simulink model "testFVOPID"  (R2020a)
settings: Solver=VariableStepAuto  StartTime=0.0  StopTime=50  RelTol=1e-3
settings Model: Creator=dell-wi  LastModifiedBy=Pio
settings DataIOCC: ReturnWorkspaceOutputs=off
settings DebuggingCC: ArithmeticOperatorsInVariantConditions=warning
settings SFSimCC: SimUseLocalCustomCode=off  CustomCodeUndefinedFunction=UseInterfaceOnly
settings RTWCC: RTWUseLocalCustomCode=off

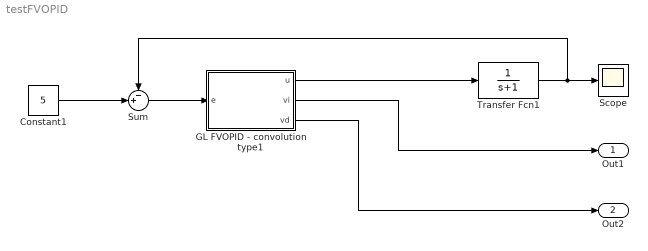
== system testFVOPID ==
  Constant1 : Constant  Value=5
  GL FVOPID - convolution type1 : Subsystem  mask{kp=1, ki=1, kd=1, sampleTime=0.01, inputBufferSize=-1, satEnab=off, satHigh=inf, satLow=-inf, integralOrderTypePopup=User defined expression, constantIntegralOrder=1, integralErrorToSetpointRatio=off, integralErrorValuesVector=[0.8, 0.6, 0.4, 0.2], integralOrderValuesVector=[1, 2, 3, 4, 5], timeDependentIntegralOrderExpression=0.1*t, derivativeOrderTypePopup=User defined expression, constantDerivativeOrder=1, derivativeErrorToSetpointRatio=off, derivativeErrorValuesVector=[0], derivativeOrderValuesVector=[1, 1], timeDependentDerivativeOrderExpression=0.1*t}
      mask prompts: kp "Proportional (P)"; ki "Integral (I)"; kd "Derivative (D)"; sampleTime "Sample time"; inputBufferSize "Input buffer size (-1 for automatically calculated)"; satEnab "Limit output"; satHigh "Upper limit"; satLow "Lower limit"; integralOrderTypePopup "Integral order type"; constantIntegralOrder "Integral order"; integralErrorToSetpointRatio "Use error/setpoint ratio"; integralErrorValuesVector "Vector of control error values"; integralOrderValuesVector "Vector of order values"; derivativeOrderTypePopup "Derivative order type"; constantDerivativeOrder "Derivative order"; derivativeErrorToSetpointRatio "Use error/setpoint ratio"; derivativeErrorValuesVector "Vector of control error values"; derivativeOrderValuesVector "Vector of order values"
      mask init:
      | % Initialize block parameters
      | fvopidToolbox.library.utils.initializeBasicModelParameters(sampleTime, inputBufferSize,'fvopidConv');
      | integralOrderTypeComboBoxValue = get_param(gcb,'integralOrderTypePopup');
      | derivativeOrderTypeComboBoxValue = get_param(gcb,'derivativeOrderTypePopup');
      | 
      | % Set order function type
      | switch integralOrderTypeComboBoxValue
      |     case 'Constant order'
      |         integralOrderType = 1;
      |     case 'Control error function'
      |         integralErrorToSetpointRatioValue = get_param(gcb,'integralErrorToSetpointRatio');
      |         if strcmp(integralErrorToSetpointRatioValue, 'on')
      |             integralOrderType = 3;
      |         else
      |             integralOrderType = 2;
      |         end
      |     otherwise
      |         integralOrderExpressionCode = get_param(gcb,'timeDependentIntegralOrderExpression');
      |         newScript = sprintf(['function y = integralTimeDependentMatlabFunction(t, e)\n'...
      |             'y = '  integralOrderExpressionCode ';\nend']);
      |         fvopidToolbox.utils.updateMatlabFunctionBlockScript('integralTimeDependentBlock', newScript,...
      |             [gcb '/integralTimeDependentSubsystem/integralTimeDependentBlock']);
      |         integralOrderType = 4;
      | end
      | 
      | switch derivativeOrderTypeComboBoxValue
      |     case 'Constant order'
      |         derivativeOrderType = 1;
      |     case 'Control error function'
      |         derivatieErrorToSetpointRatioValue = get_param(gcb,'derivativeErrorToSetpointRatio');
      |         if strcmp(derivatieErrorToSetpointRatioValue, 'on')
      |             derivativeOrderType = 3;
      |         else
      |             derivativeOrderType = 2;
      |         end
      |     otherwise
      |         derivativeOrderExpressionCode = get_param(gcb,'timeDependentDerivativeOrderExpression');
      |         newScript = sprintf(['function y = derivativeTimeDependentMatlabFunction(t, e)\n'...
      |             'y = ' derivativeOrderExpressionCode ';\nend']);
      |         fvopidToolbox.utils.updateMatlabFunctionBlockScript('derivativeTimeDependentBlock', newScript,...
      |             [gcb '/derivativeTimeDependentSubsystem/derivativeTimeDependentBlock']);
      |         derivativeOrderType = 4;
      | end
      | 
      | % Update the input ports
      | setpointInputBlock = find_system(gcb,...
      |     'LookUnderMasks','on',...
      |     'FollowLinks','on','Name','setpointInput');
      | if integralOrderType == 3 || derivativeOrderType == 3
      |     if isempty(setpointInputBlock)
      |         add_block('built-in/Inport',[gcb,'/setpointInput']);  
      |     else
      |         h = get_param([gcb '/setpointInput'], 'LineHandles'); 
      |         delete_line(h.Outport(1));
      |     end
      | 
      |     if integralOrderType == 3
      |         add_line(gcb,'setpointInput/1','integralRatioDependentSubsystem/2');
      |     end
      | 
      |     if derivativeOrderType == 3
      |         add_line(gcb,'setpointInput/1','derivativeRatioDependentSubsystem/2');
      |     end
      | else
      |     if ~isempty(setpointInputBlock)
      |         h = get_param([gcb '/setpointInput'], 'LineHandles'); 
      |         delete_line(h.Outport(1));
      |         delete_block(setpointInputBlock);
      |     end
      | end
      settings: CopyFcn=set_param(gcbh, 'LinkStatus', 'none');
      mask Callback satEnab:
      | limitOutputCheckBoxValue = get_param(gcb,'satEnab');
      | if strcmp(limitOutputCheckBoxValue, 'on')
      |    fvopidToolbox.library.utils.setMaskParameterPropertyValue('satHigh', 'MaskEnables', 'on');
      |    fvopidToolbox.library.utils.setMaskParameterPropertyValue('satLow', 'MaskEnables', 'on');
      | else
      |    fvopidToolbox.library.utils.setMaskParameterPropertyValue('satHigh', 'MaskEnables', 'off');
      |    fvopidToolbox.library.utils.setMaskParameterPropertyValue('satLow', 'MaskEnables', 'off');
      | end
      mask TypeOptions integralOrderTypePopup: Constant order | Function of control error | User defined expression
      mask Callback integralOrderTypePopup:
      | selectedComboBoxValue = get_param(gcb,'integralOrderTypePopup');
      | 
      | switch selectedComboBoxValue
      |     case 'Constant order'
      |         fvopidToolbox.library.utils.setMaskElementVisiblePropertyValue('constantIntegralOrderPanel', 'on');
      |         fvopidToolbox.library.utils.setMaskElementVisiblePropertyValue('controlErrorDependentIntegralOrderPanel', 'off');
      |         fvopidToolbox.library.utils.setMaskElementVisiblePropertyValue('timeDependentIntegralOrderPanel', 'off');
      |     case 'Control error function'
      |         fvopidToolbox.library.utils.setMaskElementVisiblePropertyValue('constantIntegralOrderPanel', 'off');
      |         fvopidToolbox.library.utils.setMaskElementVisiblePropertyValue('controlErrorDependentIntegralOrderPanel', 'on');
      |         fvopidToolbox.library.utils.setMaskElementVisiblePropertyValue('timeDependentIntegralOrderPanel', 'off');
      |     otherwise
      |         fvopidToolbox.library.utils.setMaskElementVisiblePropertyValue('constantIntegralOrderPanel', 'off');
      |         fvopidToolbox.library.utils.setMaskElementVisiblePropertyValue('controlErrorDependentIntegralOrderPanel', 'off');
      |         fvopidToolbox.library.utils.setMaskElementVisiblePropertyValue('timeDependentIntegralOrderPanel', 'on');
      | end
      mask TypeOptions derivativeOrderTypePopup: Constant order | Function of control error | User defined expression
      mask Callback derivativeOrderTypePopup:
      | selectedComboBoxValue = get_param(gcb,'derivativeOrderTypePopup');
      | 
      | switch selectedComboBoxValue
      |     case 'Constant order'
      |         fvopidToolbox.library.utils.setMaskElementVisiblePropertyValue('constantDerivativeOrderPanel', 'on');
      |         fvopidToolbox.library.utils.setMaskElementVisiblePropertyValue('controlErrorDependentDerivativeOrderPanel', 'off');
      |         fvopidToolbox.library.utils.setMaskElementVisiblePropertyValue('timeDependentDerivativeOrderPanel', 'off');
      |     case 'Control error function'
      |         fvopidToolbox.library.utils.setMaskElementVisiblePropertyValue('constantDerivativeOrderPanel', 'off');
      |         fvopidToolbox.library.utils.setMaskElementVisiblePropertyValue('controlErrorDependentDerivativeOrderPanel', 'on');
      |         fvopidToolbox.library.utils.setMaskElementVisiblePropertyValue('timeDependentDerivativeOrderPanel', 'off');
      |     otherwise
      |         fvopidToolbox.library.utils.setMaskElementVisiblePropertyValue('constantDerivativeOrderPanel', 'off');
      |         fvopidToolbox.library.utils.setMaskElementVisiblePropertyValue('controlErrorDependentDerivativeOrderPanel', 'off');
      |         fvopidToolbox.library.utils.setMaskElementVisiblePropertyValue('timeDependentDerivativeOrderPanel', 'on');
      | end
      mask DialogControl mainTab Prompt: Main
      mask DialogControl controllerParametersGroupBox Prompt: Controller parameters
      mask DialogControl outputSaturationTab Prompt: Output saturation
      mask DialogControl outputSaturationGroupBox Prompt: Output saturation
      mask DialogControl integralOrderTab Prompt: Integral order
      mask DialogControl errorDependentIntegralOrderDescription1 Prompt: Provide a vector of control error values and a vector of order vales. Vector of order values should have one element more than the vector of error. E.g. for if the vector of order values is: [e1, e2, e3] and the vector of orders is [o1, o2, o3, o4], then the orders are generated according to the following rule:
      mask DialogControl errorDependentIntegralOrderDescription2 Prompt: - order = o1 for errors > e1,
      mask DialogControl errorDependentIntegralOrderDescription3 Prompt: - order = o2 for e2 < error <= e1,
      mask DialogControl errorDependentIntegralOrderDescription4 Prompt: - order = o3 for e3 < error <= e2,
      mask DialogControl errorDependentIntegralOrderDescription5 Prompt: - order = o4 for error < e3.
      mask DialogControl timeDependentIntegralOrderDescription1 Prompt: Insert short expression which returns value of order as a function of time (t) and/or control error (e), e.g.: '2*t + e' (where 't' is current simulation time and 'e' is current value of the control error).
      mask DialogControl derivativeOrderTab Prompt: Derivative order
      mask DialogControl errorDependentDerivativeOrderDescription1 Prompt: Provide a vector of control error values and a vector of order vales. Vector of order values should have one element more than the vector of error. E.g. for if the vector of order values is: [e1, e2, e3] and the vector of orders is [o1, o2, o3, o4], then the orders are generated according to the following rule:
      mask DialogControl errorDependentDerivativeOrderDescription2 Prompt: - order = o1 for errors > e1,
      mask DialogControl errorDependentDerivativeOrderDescription3 Prompt: - order = o2 for e2 < error <= e1,
      mask DialogControl errorDependentDerivativeOrderDescription4 Prompt: - order = o3 for e3 < error <= e2,
      mask DialogControl errorDependentDerivativeOrderDescription5 Prompt: - order = o4 for error < e3.
      mask DialogControl timeDependentDerivativeOrderDescription1 Prompt: Insert short expression which returns value of order as a function of time (t) and/or control error (e), e.g.: '2*t + e' (where 't' is current simulation time and 'e' is current value of the control error).
  Scope : Scope
  Sum : Sum  Inputs=-+|
  Transfer Fcn1 : TransferFcn  Denominator=[1 1]
  Out1 : Outport
  Out2 : Outport  Port=2
  wires:
  Constant1/1 -> Sum/2
  Transfer Fcn1/1 -> Sum/1, Scope/1
  GL FVOPID - convolution type1/1(u) -> Transfer Fcn1/1
  Sum/1 -> GL FVOPID - convolution type1/1(e)
  GL FVOPID - convolution type1/2(vi) -> Out1/1
  GL FVOPID - convolution type1/3(vd) -> Out2/1

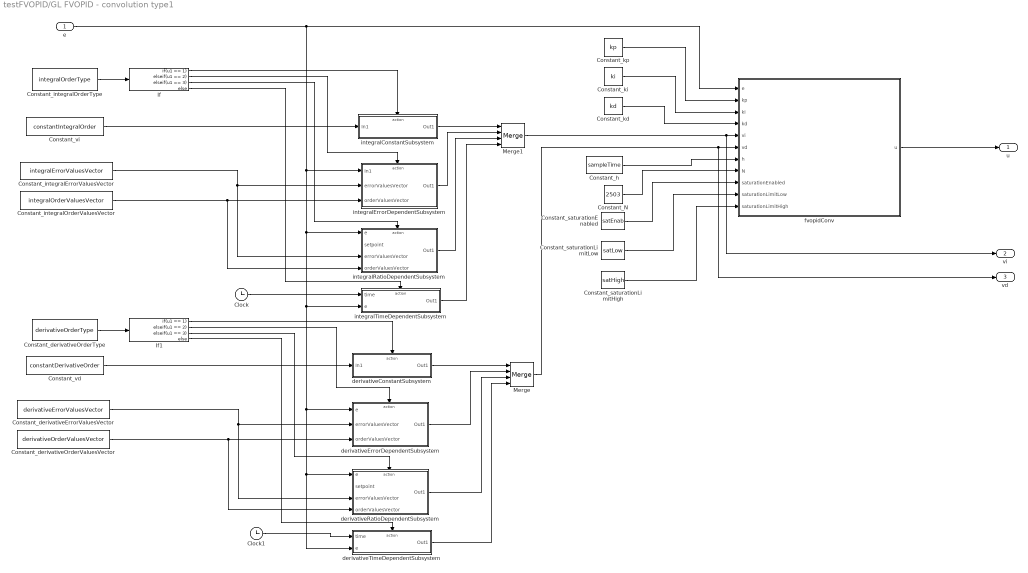
== system testFVOPID/GL FVOPID - convolution type1 ==
  e : Inport
  Clock : Clock
  Clock1 : Clock
  Constant_N : Constant  Value=2503
  Constant_derivativeErrorValuesVector : Constant  Value=derivativeErrorValuesVector
  Constant_derivativeOrderType : Constant  Value=derivativeOrderType
  Constant_derivativeOrderValuesVector : Constant  Value=derivativeOrderValuesVector
  Constant_h : Constant  Value=sampleTime
  Constant_integralErrorValuesVector : Constant  Value=integralErrorValuesVector
  Constant_integralOrderType : Constant  Value=integralOrderType
  Constant_integralOrderValuesVector : Constant  Value=integralOrderValuesVector
  Constant_kd : Constant  Value=kd
  Constant_ki : Constant  Value=ki
  Constant_kp : Constant  Value=kp
  Constant_saturationEnabled : Constant  Value=satEnab
  Constant_saturationLimitHigh : Constant  Value=satHigh
  Constant_saturationLimitLow : Constant  Value=satLow
  Constant_vd : Constant  Value=constantDerivativeOrder
  Constant_vi : Constant  Value=constantIntegralOrder
  If : If  IfExpression=u1 == 1  ElseIfExpressions=u1 == 2, u1 == 3
  If1 : If  IfExpression=u1 == 1  ElseIfExpressions=u1 == 2, u1 == 3
  Merge : Merge  Inputs=4
  Merge1 : Merge  Inputs=4
  derivativeConstantSubsystem : Subsystem  TreatAsAtomicUnit=on
  derivativeErrorDependentSubsystem : Subsystem  TreatAsAtomicUnit=on
  derivativeRatioDependentSubsystem : Subsystem  TreatAsAtomicUnit=on
  derivativeTimeDependentSubsystem : Subsystem  TreatAsAtomicUnit=on
  fvopidConv : MATLAB Function  TreatAsAtomicUnit=on  SystemSampleTime=0.01
  integralConstantSubsystem : Subsystem  TreatAsAtomicUnit=on
  integralErrorDependentSubsystem : Subsystem  TreatAsAtomicUnit=on
  integralRatioDependentSubsystem : Subsystem  TreatAsAtomicUnit=on
  integralTimeDependentSubsystem : Subsystem  TreatAsAtomicUnit=on
  u : Outport  VectorParamsAs1DForOutWhenUnconnected=off
  vi : Outport  Port=2  VectorParamsAs1DForOutWhenUnconnected=off
  vd : Outport  Port=3  VectorParamsAs1DForOutWhenUnconnected=off
  wires:
  Constant_saturationLimitHigh/1 -> fvopidConv/11(saturationLimitHigh)
  e/1 -> integralErrorDependentSubsystem/1(In1), integralRatioDependentSubsystem/1(e), integralTimeDependentSubsystem/2(e), derivativeTimeDependentSubsystem/2(e), derivativeRatioDependentSubsystem/1(e), derivativeErrorDependentSubsystem/1(e), fvopidConv/1(e)
  Constant_N/1 -> fvopidConv/8(N)
  Constant_h/1 -> fvopidConv/7(h)
  Constant_kp/1 -> fvopidConv/2(kp)
  Constant_saturationLimitLow/1 -> fvopidConv/10(saturationLimitLow)
  fvopidConv/1(u) -> u/1
  Constant_saturationEnabled/1 -> fvopidConv/9(saturationEnabled)
  Constant_kd/1 -> fvopidConv/4(kd)
  Constant_ki/1 -> fvopidConv/3(ki)
  Merge1/1 -> vi/1, fvopidConv/5(vi)
  Merge/1 -> vd/1, fvopidConv/6(vd)
  Constant_integralOrderType/1 -> If/1
  integralConstantSubsystem/1(Out1) -> Merge1/1
  integralErrorDependentSubsystem/1(Out1) -> Merge1/2
  Constant_vi/1 -> integralConstantSubsystem/1(In1)
  If/1 -> integralConstantSubsystem/Action
  Constant_integralErrorValuesVector/1 -> integralErrorDependentSubsystem/2(errorValuesVector), integralRatioDependentSubsystem/3(errorValuesVector)
  Constant_integralOrderValuesVector/1 -> integralRatioDependentSubsystem/4(orderValuesVector), integralErrorDependentSubsystem/3(orderValuesVector)
  integralRatioDependentSubsystem/1(Out1) -> Merge1/3
  If/2 -> integralErrorDependentSubsystem/Action
  If/4 -> integralTimeDependentSubsystem/Action
  Constant_derivativeOrderType/1 -> If1/1
  Constant_vd/1 -> derivativeConstantSubsystem/1(In1)
  derivativeConstantSubsystem/1(Out1) -> Merge/1
  If1/1 -> derivativeConstantSubsystem/Action
  If1/2 -> derivativeErrorDependentSubsystem/Action
  Constant_derivativeErrorValuesVector/1 -> derivativeRatioDependentSubsystem/3(errorValuesVector), derivativeErrorDependentSubsystem/2(errorValuesVector)
  Constant_derivativeOrderValuesVector/1 -> derivativeRatioDependentSubsystem/4(orderValuesVector), derivativeErrorDependentSubsystem/3(orderValuesVector)
  derivativeErrorDependentSubsystem/1(Out1) -> Merge/2
  derivativeRatioDependentSubsystem/1(Out1) -> Merge/3
  Clock/1 -> integralTimeDependentSubsystem/1(time)
  integralTimeDependentSubsystem/1(Out1) -> Merge1/4
  If/3 -> integralRatioDependentSubsystem/Action
  If1/3 -> derivativeRatioDependentSubsystem/Action
  If1/4 -> derivativeTimeDependentSubsystem/Action
  Clock1/1 -> derivativeTimeDependentSubsystem/1(time)
  derivativeTimeDependentSubsystem/1(Out1) -> Merge/4

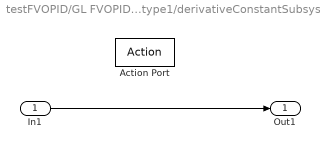
== system testFVOPID/GL FVOPID - convolution type1/derivativeConstantSubsystem ==
  In1 : Inport
  Action Port : ActionPort  ActionPortLabel=if(u1 == 1)
  Out1 : Outport  VectorParamsAs1DForOutWhenUnconnected=off
  wires:
  In1/1 -> Out1/1

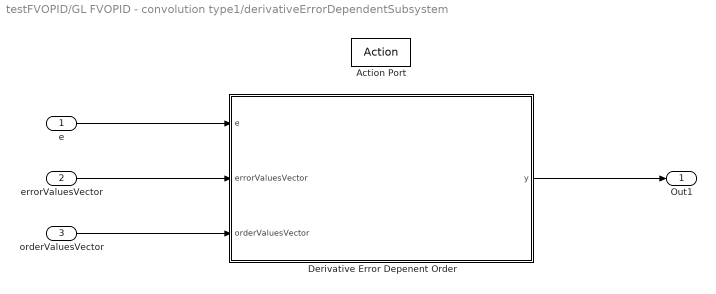
== system testFVOPID/GL FVOPID - convolution type1/derivativeErrorDependentSubsystem ==
  e : Inport
  errorValuesVector : Inport  Port=2
  orderValuesVector : Inport  Port=3
  Action Port : ActionPort  ActionPortLabel=elseif(u1 == 2)
  Derivative Error Depenent Order : MATLAB Function  TreatAsAtomicUnit=on
  Out1 : Outport  VectorParamsAs1DForOutWhenUnconnected=off
  wires:
  e/1 -> Derivative Error Depenent Order/1(e)
  Derivative Error Depenent Order/1(y) -> Out1/1
  errorValuesVector/1 -> Derivative Error Depenent Order/2(errorValuesVector)
  orderValuesVector/1 -> Derivative Error Depenent Order/3(orderValuesVector)

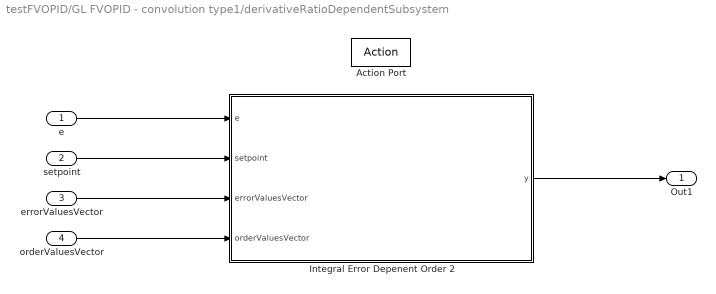
== system testFVOPID/GL FVOPID - convolution type1/derivativeRatioDependentSubsystem ==
  e : Inport
  setpoint : Inport  Port=2
  errorValuesVector : Inport  Port=3
  orderValuesVector : Inport  Port=4
  Action Port : ActionPort  ActionPortLabel=elseif( u1 == 3)
  Integral Error Depenent Order 2 : MATLAB Function  TreatAsAtomicUnit=on
  Out1 : Outport  VectorParamsAs1DForOutWhenUnconnected=off
  wires:
  e/1 -> Integral Error Depenent Order 2/1(e)
  Integral Error Depenent Order 2/1(y) -> Out1/1
  errorValuesVector/1 -> Integral Error Depenent Order 2/3(errorValuesVector)
  orderValuesVector/1 -> Integral Error Depenent Order 2/4(orderValuesVector)
  setpoint/1 -> Integral Error Depenent Order 2/2(setpoint)

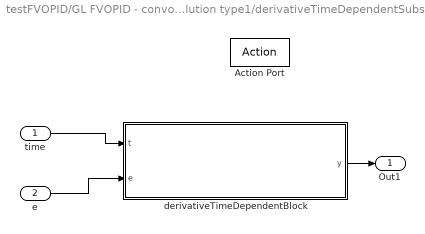
== system testFVOPID/GL FVOPID - convolution type1/derivativeTimeDependentSubsystem ==
  time : Inport
  e : Inport  Port=2
  Action Port : ActionPort  ActionPortLabel=else
  derivativeTimeDependentBlock : MATLAB Function  TreatAsAtomicUnit=on
  Out1 : Outport  VectorParamsAs1DForOutWhenUnconnected=off
  wires:
  time/1 -> derivativeTimeDependentBlock/1(t)
  derivativeTimeDependentBlock/1(y) -> Out1/1
  e/1 -> derivativeTimeDependentBlock/2(e)

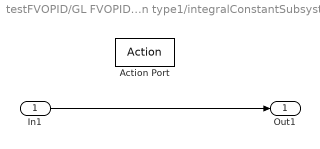
== system testFVOPID/GL FVOPID - convolution type1/integralConstantSubsystem ==
  In1 : Inport
  Action Port : ActionPort  ActionPortLabel=if(u1 == 1)
  Out1 : Outport  VectorParamsAs1DForOutWhenUnconnected=off
  wires:
  In1/1 -> Out1/1

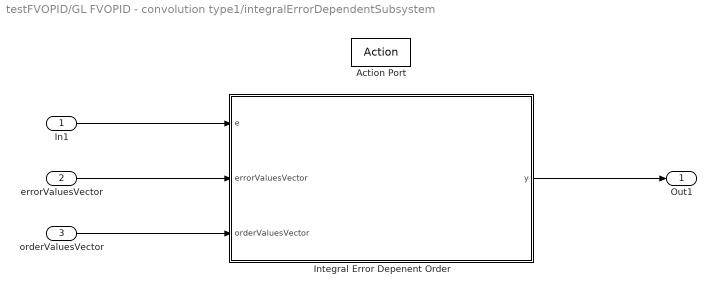
== system testFVOPID/GL FVOPID - convolution type1/integralErrorDependentSubsystem ==
  In1 : Inport
  errorValuesVector : Inport  Port=2
  orderValuesVector : Inport  Port=3
  Action Port : ActionPort  ActionPortLabel=elseif(u1 == 2)
  Integral Error Depenent Order : MATLAB Function  TreatAsAtomicUnit=on
  Out1 : Outport  VectorParamsAs1DForOutWhenUnconnected=off
  wires:
  In1/1 -> Integral Error Depenent Order/1(e)
  Integral Error Depenent Order/1(y) -> Out1/1
  errorValuesVector/1 -> Integral Error Depenent Order/2(errorValuesVector)
  orderValuesVector/1 -> Integral Error Depenent Order/3(orderValuesVector)

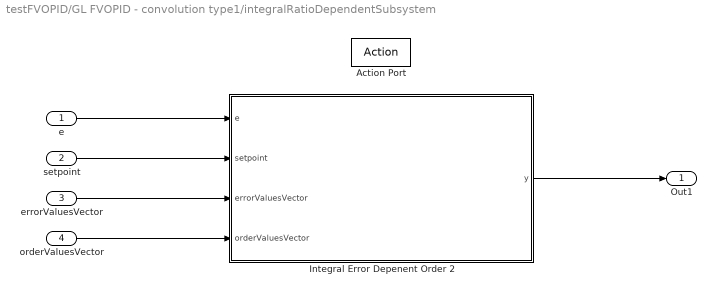
== system testFVOPID/GL FVOPID - convolution type1/integralRatioDependentSubsystem ==
  e : Inport
  setpoint : Inport  Port=2
  errorValuesVector : Inport  Port=3
  orderValuesVector : Inport  Port=4
  Action Port : ActionPort  ActionPortLabel=elseif( u1 == 3)
  Integral Error Depenent Order 2 : MATLAB Function  TreatAsAtomicUnit=on
  Out1 : Outport  VectorParamsAs1DForOutWhenUnconnected=off
  wires:
  e/1 -> Integral Error Depenent Order 2/1(e)
  Integral Error Depenent Order 2/1(y) -> Out1/1
  errorValuesVector/1 -> Integral Error Depenent Order 2/3(errorValuesVector)
  orderValuesVector/1 -> Integral Error Depenent Order 2/4(orderValuesVector)
  setpoint/1 -> Integral Error Depenent Order 2/2(setpoint)

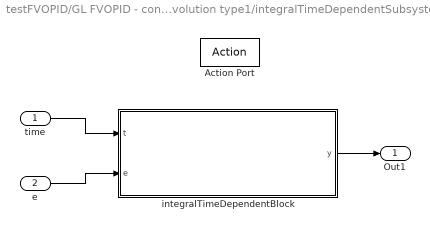
== system testFVOPID/GL FVOPID - convolution type1/integralTimeDependentSubsystem ==
  time : Inport
  e : Inport  Port=2
  Action Port : ActionPort  ActionPortLabel=else
  integralTimeDependentBlock : MATLAB Function  TreatAsAtomicUnit=on
  Out1 : Outport  VectorParamsAs1DForOutWhenUnconnected=off
  wires:
  time/1 -> integralTimeDependentBlock/1(t)
  integralTimeDependentBlock/1(y) -> Out1/1
  e/1 -> integralTimeDependentBlock/2(e)

== matlab function testFVOPID/GL FVOPID - convolution type1/derivativeErrorDependentSubsystem/Derivative Error Depenent Order ==
  data: e input; y output; errorValuesVector input; orderValuesVector input
function y = derivativeOrderFunction(e, errorValuesVector, orderValuesVector)
    y = fvopidToolbox.utils.getOrderValue(e, errorValuesVector, orderValuesVector);
end

== matlab function testFVOPID/GL FVOPID - convolution type1/derivativeRatioDependentSubsystem/Integral Error Depenent Order 2 ==
  data: e input; setpoint input; y output; errorValuesVector input; orderValuesVector input
function y = integralOrderFunction(e, setpoint, errorValuesVector, orderValuesVector)
    y = fvopidToolbox.utils.getOrderValue(e/setpoint, errorValuesVector, orderValuesVector);
end

== matlab function testFVOPID/GL FVOPID - convolution type1/derivativeTimeDependentSubsystem/derivativeTimeDependentBlock ==
  data: t input; y output; e input
function y = derivativeTimeDependentMatlabFunction(t, e)
y = 0.1*t;
end

== matlab function testFVOPID/GL FVOPID - convolution type1/fvopidConv ==
  data: e input; u output; kp input; ki input; kd input; vi input; vd input; h input; N input; saturationEnabled input; saturationLimitLow input; saturationLimitHigh input
function u = fvopidConv(e, kp, ki, kd, vi, vd, h, N, saturationEnabled, saturationLimitLow, saturationLimitHigh)
    u = fvopidToolbox.fvopid.fvopidConv(e, kp, ki, kd, vi, vd, h, N, saturationEnabled, saturationLimitLow, saturationLimitHigh);

== matlab function testFVOPID/GL FVOPID - convolution type1/integralErrorDependentSubsystem/Integral Error Depenent Order ==
  data: e input; y output; errorValuesVector input; orderValuesVector input
function y = integralOrderFunction(e, errorValuesVector, orderValuesVector)
    y = fvopidToolbox.utils.getOrderValue(e, errorValuesVector, orderValuesVector);
end

== matlab function testFVOPID/GL FVOPID - convolution type1/integralRatioDependentSubsystem/Integral Error Depenent Order 2 ==
  data: e input; setpoint input; y output; errorValuesVector input; orderValuesVector input
function y = integralOrderFunction(e, setpoint, errorValuesVector, orderValuesVector)
    y = fvopidToolbox.utils.getOrderValue(e/setpoint, errorValuesVector, orderValuesVector);
end

== matlab function testFVOPID/GL FVOPID - convolution type1/integralTimeDependentSubsystem/integralTimeDependentBlock ==
  data: t input; y output; e input
function y = integralTimeDependentMatlabFunction(t, e)
y = 0.1*t;
end
